simulink library "lib_controls"  (Simulink 7.9)
settings: Solver=ode45  SolverMode=SingleTasking  StartTime=0.0  StopTime=10.0  RelTol=1e-3
undefined symbols (not defined in the file): amb_tmp, cs_charge_deplete_bool, cs_charge_pwr, cs_charge_trq, cs_clt_tmp, cs_decel_fc_off, cs_decel_regen_threshold, cs_dl_assist_trq_threshold, cs_dl_regen_trq_threshold, cs_electric_decel_spd, cs_electric_launch_spd, cs_electric_launch_spd_hi, cs_electric_launch_spd_lo, cs_eng_min_spd, cs_eng_on_soc, cs_fc_init_state, cs_fc_max_pwr_frac, cs_fc_min_pwr_frac, cs_fc_on, cs_fc_pwr_opt, cs_fc_spd_opt, cs_fuzzy_fuel_mode, cs_hi_soc, cs_hi_trq_frac, cs_lo_soc, cs_lo_trq_frac, cs_max_gc_spd, cs_max_pwr, cs_max_pwr_fall_rate, cs_max_pwr_rise_rate, cs_mc_assist_max_frac, cs_mc_assist_min_frac, cs_mc_assist_slope, cs_mc_regen_max_frac, cs_mc_regen_min_frac, cs_mc_regen_slope, cs_mean_eff, cs_mean_eff_bool, cs_min_gc_spd, cs_min_off_time, cs_min_pwr, cs_min_trq_frac, cs_mph_avg_time, cs_off_trq_frac, cs_plot_output, cs_pwr, cs_regen_avg_time, cs_scale_factor, cs_shutoff, cs_soc_range, cs_spd, cs_target_soc, cs_trq_to_soc_factor, cvt_locus_pwr, cvt_locus_spd, cyc_mph, enable_sim_stop_distance, enable_sim_stop_max_spd, enable_sim_stop_speed, enable_sim_stop_time ... (+110)
libraries: lib_controls x124, simulink3 x18, lib_etc x1
(part 4 of 17)

== system lib_controls/<vc> conv auto Saber custom/engine control ==
  shifting : Inport
  clutch state : Inport  Port=2
  fc_spd_out_r : Inport  Port=3
  v_ave_req : Inport  Port=4
  Block NOTES : Subsystem
      mask Display: disp('Block\nNOTES')
  Constant : Constant  Value=1.1
  Constant1 : Constant  Value=vc_idle_bool
  Constant2 : Constant  Value=vc_launch_spd
  Constant3 : Constant
  Constant4 : Constant  Value=0
  Constant5 : Constant  Value=0
  Constant6 : Constant  Value=0
  Logical Operator1 : Logic
  Logical Operator2 : Logic  Operator=OR
  Logical Operator3 : Logic  Operator=OR
  Logical Operator7 : Logic
  Logical Operator8 : Logic  Inputs=3
  Memory : Memory
  Saturation : Saturate  UpperLimit=max(fc_map_spd)*fc_spd_scale  LowerLimit=vc_idle_spd*vc_idle_bool
  Switch : Switch  Threshold=eps  SaturateOnIntegerOverflow=on  InputSameDT=on
  Switch1 : Switch  Threshold=eps  SaturateOnIntegerOverflow=on  InputSameDT=on
  clutch disengaged : RelationalOperator  Operator===  InputSameDT=on
  clutch slipping or engaged : RelationalOperator  Operator=>  InputSameDT=on
  key_on : Subsystem  mask(Repeating table){@1=vc_key_on(:,1), @2=vc_key_on(:,2)}
      mask prompts: @1 "Time values:"; @2 "Output values:"
      mask help:
      | Repeating table.
      | Enter values of time and output for first cycle.
      mask init:
      | period = max(@1); t = @1; y = @2;
      mask Help: Repeats cycle given in table. Time values should be monotonically increasing.
  moving next time : RelationalOperator  Operator=>  InputSameDT=on
  not moving : RelationalOperator  Operator===  InputSameDT=on
  repeated cycle:  speed required at end of NEXT step : Subsystem  mask(Forward looking repeating table){t=cyc_mph(:,1), y=cyc_mph(:,2)}
      mask prompts: t "Time values:"; y "Output values:"
      mask help:
      | Forward looking repeating table.
      | Enter values of time and output for first cycle.
      mask init:
      | period = max(t);
      mask Help: Repeats cycle given in table with a one time step forward offset. Time values should be monotonically increasing.
  engine on : Outport
  spd command  (rad/s) : Outport  Port=2
  key on : Outport  Port=3
  wires:
  clutch state/1 -> clutch slipping or engaged/1, clutch disengaged/1
  Constant/1 -> clutch slipping or engaged/2
  Constant1/1 -> Logical Operator2/2
  clutch slipping or engaged/1 -> Logical Operator2/1
  Logical Operator1/1 -> Logical Operator3/1
  Logical Operator3/1 -> Switch1/2, Memory/1, engine on/1
  Logical Operator2/1 -> Logical Operator1/2
  Constant3/1 -> clutch disengaged/2
  v_ave_req/1 -> not moving/1
  Constant4/1 -> not moving/2
  clutch disengaged/1 -> Logical Operator8/1
  not moving/1 -> Logical Operator8/2
  moving next time/1 -> Logical Operator8/3
  shifting/1 -> Logical Operator7/1
  Logical Operator7/1 -> Logical Operator3/2
  Memory/1 -> Logical Operator7/2
  repeated cycle:  speed required at end of NEXT step/1(out_1) -> moving next time/1
  Constant5/1 -> moving next time/2
  Switch/1 -> Saturation/1
  Constant2/1 -> Switch/1
  fc_spd_out_r/1 -> Switch/3
  Logical Operator8/1 -> Switch/2
  Constant6/1 -> Switch1/3
  Switch1/1 -> spd command  (rad/s)/1
  Saturation/1 -> Switch1/1
  key_on/1(out_1) -> Logical Operator1/1, key on/1

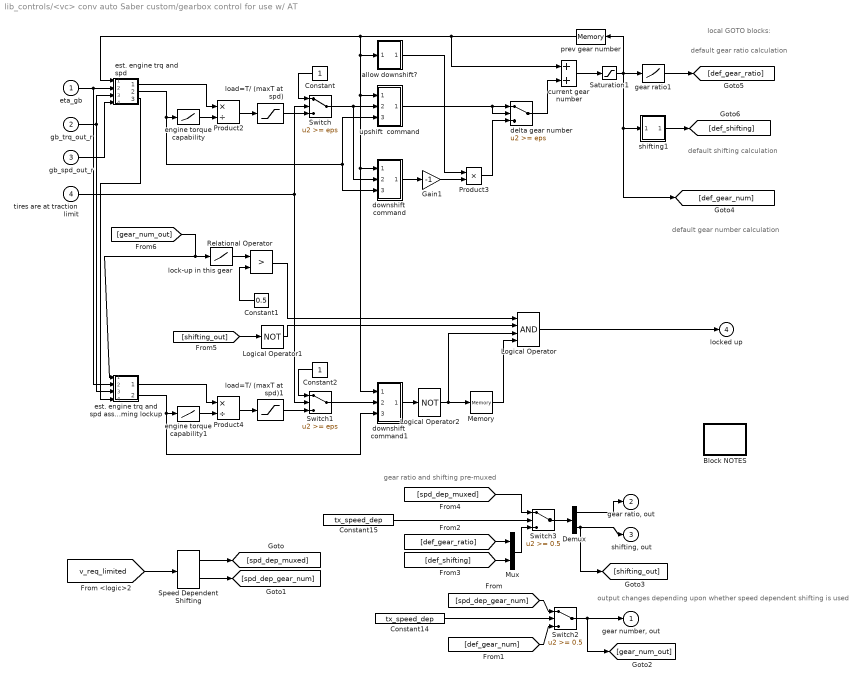
== system lib_controls/<vc> conv auto Saber custom/gearbox control for use w/ AT ==
  note: gear ratio and shifting pre-muxed
  note: output changes depending
      | upon whether speed
      | dependent shifting is used
  note: default gear number
      | calculation
  note: default shifting
      | calculation
  note: default gear ratio
      | calculation
  note: local GOTO blocks:
  eta_gb : Inport
  gb_trq_out_r : Inport  Port=2
  gb_spd_out_r : Inport  Port=3
  tires are at traction limit : Inport  Port=4
  Block NOTES : Subsystem
      mask Display: disp('Block\nNOTES')
  Constant : Constant
  Constant1 : Constant  Value=0.5
  Constant14 : Constant  Value=tx_speed_dep
  Constant15 : Constant  Value=tx_speed_dep
  Constant2 : Constant
  Demux : Demux  Outputs=2
  Gain1 : Gain  Gain=-1  SaturateOnIntegerOverflow=on  OutDataTypeStr=Inherit: Same as input  ParamDataTypeStr=Inherit: Same as input
  Logical Operator : Logic  Inputs=4
  Logical Operator1 : Logic  Operator=NOT  Inputs=1
  Logical Operator2 : Logic  Operator=NOT  Inputs=1
  Memory : Memory
  Mux : Mux  Inputs=2
  Product2 : Product  Inputs=*/  SaturateOnIntegerOverflow=on  RndMeth=Zero  InputSameDT=on  OutDataTypeStr=Inherit: Same as first input
  Product3 : Product  SaturateOnIntegerOverflow=on  RndMeth=Zero  InputSameDT=on  OutDataTypeStr=Inherit: Same as first input
  Product4 : Product  Inputs=*/  SaturateOnIntegerOverflow=on  RndMeth=Zero  InputSameDT=on  OutDataTypeStr=Inherit: Same as first input
  Relational Operator : RelationalOperator  Operator=>  InputSameDT=on
  Saturation1 : Saturate  UpperLimit=gb_gears_num  LowerLimit=1
  Speed Dependent Shifting : lib_controls/SubSystem/Speed Dependent Shifting
      settings: RTWFcnNameOpts=Auto  RTWFileNameOpts=Auto
  Switch : Switch  Threshold=eps  SaturateOnIntegerOverflow=on  InputSameDT=on
  Switch1 : Switch  Threshold=eps  SaturateOnIntegerOverflow=on  InputSameDT=on
  Switch2 : Switch  Threshold=0.5  SaturateOnIntegerOverflow=on  InputSameDT=on
  Switch3 : Switch  Threshold=0.5  SaturateOnIntegerOverflow=on  InputSameDT=on
  allow downshift? : Subsystem
  current gear number : Sum  SaturateOnIntegerOverflow=on  InputSameDT=on  OutDataTypeStr=Inherit: Same as first input
  delta gear number : Switch  Threshold=eps  SaturateOnIntegerOverflow=on  InputSameDT=on
  downshift  command : Subsystem
  downshift  command1 : Subsystem
  engine torque capability : Lookup  InputValues=fc_map_spd*fc_spd_scale  Table=fc_max_trq*fc_trq_scale+eps  SaturateOnIntegerOverflow=on
  engine torque capability1 : Lookup  InputValues=fc_map_spd*fc_spd_scale  Table=fc_max_trq*fc_trq_scale+eps  SaturateOnIntegerOverflow=on
  est. engine trq and spd : Subsystem
  est. engine trq and spd assuming lockup : Subsystem
  gear ratio1 : Lookup  InputValues=[1:length(gb_ratio)]  Table=gb_ratio  SaturateOnIntegerOverflow=on
  load=T/ (maxT at spd) : Saturate  UpperLimit=1  LowerLimit=-1
  load=T/ (maxT at spd)1 : Saturate  UpperLimit=1  LowerLimit=-1
  lock-up in this gear : Lookup  InputValues=[1:length(htc_lockup)]  Table=htc_lockup  SaturateOnIntegerOverflow=on
  prev gear number : Memory  X0=gb_num_init
  shifting1 : Subsystem
  upshift  command : Subsystem
  "gear number, out" : Outport  InitialOutput=0
  "gear ratio, out" : Outport  Port=2  InitialOutput=0
  "shifting, out" : Outport  Port=3  InitialOutput=0
  locked up : Outport  Port=4  InitialOutput=0
  wires:
  downshift  command1/1(command) -> Logical Operator2/1
  load=T/ (maxT at spd)1/1 -> Switch1/3
  Memory/1 -> Logical Operator/4
  Switch1/1 -> downshift  command1/2(engine load)
  Logical Operator/1 -> locked up/1
  Gain1/1 -> Product3/2
  upshift  command/1(command) -> delta gear number/1, delta gear number/2
  Switch/1 -> upshift  command/2(engine load), downshift  command/2(engine load)
  Logical Operator2/1 -> Memory/1, Logical Operator/3
  est. engine trq and spd assuming lockup/2(est eng spd (rad/s)) -> downshift  command1/3(engine speed), engine torque capability1/1
  est. engine trq and spd/3(gb_spd_in_est (rad/s)1) -> est. engine trq and spd assuming lockup/4(gb_spd_in_est)
  tires are at traction limit/1 -> Switch/2, Switch1/2
  gb_trq_out_r/1 -> est. engine trq and spd assuming lockup/3(gb_trq_out_r), est. engine trq and spd/3(gb_trq_out_r)
  eta_gb/1 -> est. engine trq and spd assuming lockup/2(" prev eta_gb"), est. engine trq and spd/2(" prev eta_gb")
  est. engine trq and spd assuming lockup/1(est eng trq (Nm)) -> Product4/1
  engine torque capability1/1 -> Product4/2
  Product4/1 -> load=T/ (maxT at spd)1/1
  Constant2/1 -> Switch1/1
  Logical Operator1/1 -> Logical Operator/2
  downshift  command/1(command) -> Gain1/1
  load=T/ (maxT at spd)/1 -> Switch/3
  est. engine trq and spd/1(est eng trq (Nm)) -> Product2/1
  engine torque capability/1 -> Product2/2
  current gear number/1 -> Saturation1/1
  Product3/1 -> delta gear number/3
  allow downshift?/1(allow shift) -> Product3/1
  delta gear number/1 -> current gear number/2
  Product2/1 -> load=T/ (maxT at spd)/1
  Constant/1 -> Switch/1
  Saturation1/1 -> gear ratio1/1, prev gear number/1, shifting1/1(gear number), [def_gear_num]
  prev gear number/1 -> est. engine trq and spd/1(prev gear number), allow downshift?/1(prev gearnum), downshift  command1/1(prev gear number), downshift  command/1(prev gear number), upshift  command/1(prev gear number), current gear number/1
  gb_spd_out_r/1 -> est. engine trq and spd/4(gb_spd_out_r)
  est. engine trq and spd/2(est eng spd (rad/s)) -> engine torque capability/1, upshift  command/3(engine speed), downshift  command/3(engine speed)
  Constant15/1 -> Switch3/2
  [spd_dep_muxed] -> Switch3/1
  Mux/1 -> Switch3/3
  [def_gear_ratio] -> Mux/1
  [def_shifting] -> Mux/2
  Switch3/1 -> Demux/1
  Demux/1 -> "gear ratio, out"/1
  Constant14/1 -> Switch2/2
  [spd_dep_gear_num] -> Switch2/1
  [def_gear_num] -> Switch2/3
  [v_req_limited] -> Speed Dependent Shifting/1
  Speed Dependent Shifting/1 -> [spd_dep_muxed]
  Speed Dependent Shifting/2 -> [spd_dep_gear_num]
  Switch2/1 -> "gear number, out"/1, [gear_num_out]
  Demux/2 -> "shifting, out"/1, [shifting_out]
  [shifting_out] -> Logical Operator1/1
  [gear_num_out] -> lock-up in this gear/1, est. engine trq and spd assuming lockup/1(new gear number)
  Relational Operator/1 -> Logical Operator/1
  lock-up in this gear/1 -> Relational Operator/1
  Constant1/1 -> Relational Operator/2
  gear ratio1/1 -> [def_gear_ratio]
  shifting1/1(out_1) -> [def_shifting]

== system lib_controls/<vc> conv cvt/clutch control ==
  shifting : Inport
  gb_trq_in_r : Inport  Port=2
  gb_spd_in_r : Inport  Port=3
  Block NOTES : Subsystem
      mask Display: disp('Block\nNOTES')
  Constant : Constant  Value=1e-3
  Constant1 : Constant  Value=vc_clutch_bool
  Constant2 : Constant  Value=vc_idle_spd
  Constant3 : Constant  Value=1e-3
  Constant4 : Constant  Value=vc_launch_spd
  Constant5 : Constant  Value=2.5
  Fcn: 1 if clutch disengaged 2 if clutch slipping 3 if clutch engaged : Fcn  Expr=u[1]+2*u[2]*(1-u[1])*(1-u[3])+3*u[3]*(1-u[1])
  Logical Operator : Logic
  Logical Operator1 : Logic  Operator=OR
  Memory : Memory  X0=1+(2*(cyc_mph(1,2)>0))
  Mux : Mux  Inputs=3
  Relational Operator : RelationalOperator  Operator=<=  InputSameDT=on
  Relational Operator1 : RelationalOperator  Operator=<  InputSameDT=on
  Relational Operator2 : RelationalOperator  Operator=>  InputSameDT=on
  Relational Operator3 : RelationalOperator  Operator=<  InputSameDT=on
  clutch disengaged : Logic  Operator=OR
  clutch engaged : Logic  Operator=NOR
  clutch slipping : Logic  Inputs=3
  clutch was NOT fully engaged during last time step : RelationalOperator  Operator=<  InputSameDT=on
  clutch state : Outport
  wires:
  Relational Operator1/1 -> Logical Operator1/2
  Constant2/1 -> Relational Operator1/2
  gb_spd_in_r/1 -> Relational Operator1/1, Relational Operator3/1
  Mux/1 -> Fcn: 1 if clutch disengaged 2 if clutch slipping 3 if clutch engaged/1
  clutch engaged/1 -> Mux/3
  clutch disengaged/1 -> clutch engaged/1, Mux/1
  Fcn: 1 if clutch disengaged 2 if clutch slipping 3 if clutch engaged/1 -> clutch state/1, Memory/1
  Constant3/1 -> Relational Operator2/2
  Relational Operator2/1 -> clutch slipping/1
  clutch slipping/1 -> clutch engaged/2, Mux/2
  Constant4/1 -> Relational Operator3/2
  Relational Operator3/1 -> clutch slipping/2
  Memory/1 -> clutch was NOT fully engaged during last time step/1
  Constant5/1 -> clutch was NOT fully engaged during last time step/2
  clutch was NOT fully engaged during last time step/1 -> clutch slipping/3
  Constant1/1 -> Logical Operator1/1
  Constant/1 -> Relational Operator/2
  Relational Operator/1 -> Logical Operator/1
  Logical Operator1/1 -> Logical Operator/2
  gb_trq_in_r/1 -> Relational Operator/1, Relational Operator2/1
  Logical Operator/1 -> clutch disengaged/2
  shifting/1 -> clutch disengaged/1

== system lib_controls/<vc> conv cvt/config traction control ==
  time-average vehicle speed  req'd (m/s) : Inport
  vehicle speed at beginning of time  step (m/s) : Inport  Port=2
  total tractive force req'd (N) : Inport  Port=3
  traction control 2 axle : lib_controls/SubSystem/traction control 2 axle
  req'd force (N) : Outport
  req'd speed (m/s) : Outport  Port=2
  weight on front axle (N) : Outport  Port=3
  weight on rear axle (N) : Outport  Port=4
  front/total  traction ratio : Outport  Port=5
  wires:
  time-average vehicle speed  req'd (m/s)/1 -> traction control 2 axle/1
  vehicle speed at beginning of time  step (m/s)/1 -> traction control 2 axle/2
  total tractive force req'd (N)/1 -> traction control 2 axle/3
  traction control 2 axle/1 -> req'd force (N)/1
  traction control 2 axle/2 -> req'd speed (m/s)/1
  traction control 2 axle/3 -> weight on front axle (N)/1
  traction control 2 axle/4 -> weight on rear axle (N)/1
  traction control 2 axle/5 -> front/total  traction ratio/1

== system lib_controls/<vc> conv cvt/cvt control ==
  cvt_trq_out_r : Inport
  cvt_spd_out_r : Inport  Port=2
  prev. Pout/Pin : Inport  Port=3
  tires are at traction limit : Inport  Port=4
  Block NOTES : Subsystem
      mask Display: disp('Block\nNOTES')
  Constant1 : Constant  Value=eps
  Constant2 : Constant  Value=eps
  Product : Product  Inputs=**/  SaturateOnIntegerOverflow=on  RndMeth=Zero  InputSameDT=on  OutDataTypeStr=Inherit: Same as first input
  Product1 : Product  Inputs=*/  SaturateOnIntegerOverflow=on  RndMeth=Zero  InputSameDT=on  OutDataTypeStr=Inherit: Same as first input
  Saturation1 : Saturate  UpperLimit=max(gb_ratio)  LowerLimit=min(gb_ratio)
  Saturation2 : Saturate  UpperLimit=max(cvt_locus_pwr)*fc_trq_scale*fc_spd_scale  LowerLimit=min(cvt_locus_pwr)*fc_trq_scale*fc_spd_scale
  Sum : Sum  SaturateOnIntegerOverflow=on  InputSameDT=on  OutDataTypeStr=Inherit: Same as first input
  Terminator : Terminator
  desired engine speed : Lookup  InputValues=cvt_locus_pwr*fc_trq_scale*fc_spd_scale  Table=cvt_locus_spd*fc_spd_scale+eps  SaturateOnIntegerOverflow=on
  est. engine power : Sum  SaturateOnIntegerOverflow=on  InputSameDT=on  OutDataTypeStr=Inherit: Same as first input
  output speed : Sum  SaturateOnIntegerOverflow=on  InputSameDT=on  OutDataTypeStr=Inherit: Same as first input
  "pulley ratio " : Outport  InitialOutput=0
  wires:
  output speed/1 -> Product1/2
  Constant1/1 -> output speed/2
  Product/1 -> est. engine power/2
  desired engine speed/1 -> Product1/1
  est. engine power/1 -> Saturation2/1
  Product1/1 -> Saturation1/1
  Saturation2/1 -> desired engine speed/1
  [acc_mech_pwr_est] -> est. engine power/1
  cvt_spd_out_r/1 -> output speed/1, Product/2
  cvt_trq_out_r/1 -> Product/1
  prev. Pout/Pin/1 -> Sum/1
  Sum/1 -> Product/3
  Constant2/1 -> Sum/2
  tires are at traction limit/1 -> Terminator/1
  Saturation1/1 -> "pulley ratio "/1

== system lib_controls/<vc> conv cvt/engine control ==
  clutch state : Inport
  shifting : Inport  Port=2
  fc_spd_out_r : Inport  Port=3
  v_ave_req : Inport  Port=4
  Block NOTES : Subsystem
      mask Display: disp('Block\nNOTES')
  Constant : Constant  Value=1.1
  Constant1 : Constant  Value=vc_idle_bool
  Constant2 : Constant  Value=vc_launch_spd
  Constant3 : Constant
  Constant4 : Constant  Value=0
  Constant5 : Constant  Value=0
  Constant6 : Constant  Value=0
  Logical Operator1 : Logic
  Logical Operator2 : Logic  Operator=OR
  Logical Operator3 : Logic  Operator=OR
  Logical Operator7 : Logic
  Logical Operator8 : Logic  Inputs=3
  Memory : Memory
  Saturation : Saturate  UpperLimit=max(fc_map_spd)*fc_spd_scale  LowerLimit=vc_idle_spd*vc_idle_bool
  Switch : Switch  Threshold=eps  SaturateOnIntegerOverflow=on  InputSameDT=on
  Switch1 : Switch  Threshold=eps  SaturateOnIntegerOverflow=on  InputSameDT=on
  clutch disengaged : RelationalOperator  Operator===  InputSameDT=on
  clutch slipping or engaged : RelationalOperator  Operator=>  InputSameDT=on
  key_on : Subsystem  mask(Repeating table){t=vc_key_on(:,1), y=vc_key_on(:,2)}
      mask prompts: t "Time values:"; y "Output values:"
      mask help:
      | Repeating table.
      | Enter values of time and output for first cycle.
      mask init:
      | period = max(t);
      mask Help: Repeats cycle given in table. Time values should be monotonically increasing.
  moving next time : RelationalOperator  Operator=>  InputSameDT=on
  not moving : RelationalOperator  Operator===  InputSameDT=on
  repeated cycle:  speed required at end of NEXT step : Subsystem  mask(Forward looking repeating table){t=cyc_mph(:,1), y=cyc_mph(:,2)}
      mask prompts: t "Time values:"; y "Output values:"
      mask help:
      | Forward looking repeating table.
      | Enter values of time and output for first cycle.
      mask init:
      | period = max(t);
      mask Help: Repeats cycle given in table with a one time step forward offset. Time values should be monotonically increasing.
  engine on : Outport
  spd command  (rad/s) : Outport  Port=2
  key on : Outport  Port=3
  wires:
  clutch slipping or engaged/1 -> Logical Operator2/1
  Constant/1 -> clutch slipping or engaged/2
  Constant1/1 -> Logical Operator2/2
  clutch state/1 -> clutch slipping or engaged/1, clutch disengaged/1
  Logical Operator1/1 -> Logical Operator3/1
  Logical Operator3/1 -> Switch1/2, Memory/1, engine on/1
  Logical Operator2/1 -> Logical Operator1/2
  key_on/1(out_1) -> Logical Operator1/1, key on/1
  Memory/1 -> Logical Operator7/2
  shifting/1 -> Logical Operator7/1
  Logical Operator7/1 -> Logical Operator3/2
  Constant6/1 -> Switch1/3
  Switch1/1 -> spd command  (rad/s)/1
  Saturation/1 -> Switch1/1
  Constant3/1 -> clutch disengaged/2
  v_ave_req/1 -> not moving/1
  Switch/1 -> Saturation/1
  Constant4/1 -> not moving/2
  repeated cycle:  speed required at end of NEXT step/1(out_1) -> moving next time/1
  Constant5/1 -> moving next time/2
  clutch disengaged/1 -> Logical Operator8/1
  not moving/1 -> Logical Operator8/2
  moving next time/1 -> Logical Operator8/3
  Constant2/1 -> Switch/1
  fc_spd_out_r/1 -> Switch/3
  Logical Operator8/1 -> Switch/2

== system lib_controls/<vc> conv cvt Saber custom/clutch control ==
  shifting : Inport
  gb_trq_in_r : Inport  Port=2
  gb_spd_in_r : Inport  Port=3
  Block NOTES : Subsystem
      mask Display: disp('Block\nNOTES')
  Constant : Constant  Value=1e-3
  Constant1 : Constant  Value=vc_clutch_bool
  Constant2 : Constant  Value=vc_idle_spd
  Constant3 : Constant  Value=1e-3
  Constant4 : Constant  Value=vc_launch_spd
  Constant5 : Constant  Value=2.5
  Fcn: 1 if clutch disengaged 2 if clutch slipping 3 if clutch engaged : Fcn  Expr=u[1]+2*u[2]*(1-u[1])*(1-u[3])+3*u[3]*(1-u[1])
  Logical Operator : Logic
  Logical Operator1 : Logic  Operator=OR
  Memory : Memory  X0=1+(2*(cyc_mph(1,2)>0))
  Mux : Mux  Inputs=3
  Relational Operator : RelationalOperator  Operator=<=  InputSameDT=on
  Relational Operator1 : RelationalOperator  Operator=<  InputSameDT=on
  Relational Operator2 : RelationalOperator  Operator=>  InputSameDT=on
  Relational Operator3 : RelationalOperator  Operator=<  InputSameDT=on
  clutch disengaged : Logic  Operator=OR
  clutch engaged : Logic  Operator=NOR
  clutch slipping : Logic  Inputs=3
  clutch was NOT fully engaged during last time step : RelationalOperator  Operator=<  InputSameDT=on
  clutch state : Outport
  wires:
  shifting/1 -> clutch disengaged/1
  Logical Operator/1 -> clutch disengaged/2
  gb_trq_in_r/1 -> Relational Operator2/1, Relational Operator/1
  Logical Operator1/1 -> Logical Operator/2
  Relational Operator/1 -> Logical Operator/1
  Constant/1 -> Relational Operator/2
  Constant1/1 -> Logical Operator1/1
  clutch was NOT fully engaged during last time step/1 -> clutch slipping/3
  Constant5/1 -> clutch was NOT fully engaged during last time step/2
  Memory/1 -> clutch was NOT fully engaged during last time step/1
  Relational Operator3/1 -> clutch slipping/2
  Constant4/1 -> Relational Operator3/2
  clutch slipping/1 -> Mux/2, clutch engaged/2
  Relational Operator2/1 -> clutch slipping/1
  Constant3/1 -> Relational Operator2/2
  Fcn: 1 if clutch disengaged 2 if clutch slipping 3 if clutch engaged/1 -> Memory/1, clutch state/1
  clutch disengaged/1 -> Mux/1, clutch engaged/1
  clutch engaged/1 -> Mux/3
  Mux/1 -> Fcn: 1 if clutch disengaged 2 if clutch slipping 3 if clutch engaged/1
  gb_spd_in_r/1 -> Relational Operator3/1, Relational Operator1/1
  Constant2/1 -> Relational Operator1/2
  Relational Operator1/1 -> Logical Operator1/2

== system lib_controls/<vc> conv cvt Saber custom/config traction control ==
  time-average vehicle speed  req'd (m/s) : Inport
  vehicle speed at beginning of time  step (m/s) : Inport  Port=2
  total tractive force req'd (N) : Inport  Port=3
  traction control 2 axle : lib_controls/SubSystem/traction control 2 axle
      settings: RTWFcnNameOpts=Auto  RTWFileNameOpts=Auto
  req'd force (N) : Outport
  req'd speed (m/s) : Outport  Port=2
  weight on front axle (N) : Outport  Port=3
  weight on rear axle (N) : Outport  Port=4
  front/total  traction ratio : Outport  Port=5
  wires:
  time-average vehicle speed  req'd (m/s)/1 -> traction control 2 axle/1
  vehicle speed at beginning of time  step (m/s)/1 -> traction control 2 axle/2
  total tractive force req'd (N)/1 -> traction control 2 axle/3
  traction control 2 axle/1 -> req'd force (N)/1
  traction control 2 axle/2 -> req'd speed (m/s)/1
  traction control 2 axle/3 -> weight on front axle (N)/1
  traction control 2 axle/4 -> weight on rear axle (N)/1
  traction control 2 axle/5 -> front/total  traction ratio/1

== system lib_controls/<vc> conv cvt Saber custom/cvt control ==
  cvt_trq_out_r : Inport
  cvt_spd_out_r : Inport  Port=2
  prev. Pout/Pin : Inport  Port=3
  tires are at traction limit : Inport  Port=4
  Block NOTES : Subsystem
      mask Display: disp('Block\nNOTES')
  Constant1 : Constant  Value=eps
  Constant2 : Constant  Value=eps
  Product : Product  Inputs=**/  SaturateOnIntegerOverflow=on  RndMeth=Zero  InputSameDT=on  OutDataTypeStr=Inherit: Same as first input
  Product1 : Product  Inputs=*/  SaturateOnIntegerOverflow=on  RndMeth=Zero  InputSameDT=on  OutDataTypeStr=Inherit: Same as first input
  Saturation1 : Saturate  UpperLimit=max(gb_ratio)  LowerLimit=min(gb_ratio)
  Saturation2 : Saturate  UpperLimit=max(cvt_locus_pwr)*fc_trq_scale*fc_spd_scale  LowerLimit=min(cvt_locus_pwr)*fc_trq_scale*fc_spd_scale
  Sum : Sum  SaturateOnIntegerOverflow=on  InputSameDT=on  OutDataTypeStr=Inherit: Same as first input
  Terminator : Terminator
  accessories (Nm) : lib_controls/<vc> conv Saber custom/gearbox  control/accessories (Nm)
      settings: RTWFcnNameOpts=Auto  RTWFileNameOpts=Auto
  desired engine speed : Lookup  InputValues=cvt_locus_pwr*fc_trq_scale*fc_spd_scale  Table=cvt_locus_spd*fc_spd_scale+eps  SaturateOnIntegerOverflow=on
  est. engine power : Sum  SaturateOnIntegerOverflow=on  InputSameDT=on  OutDataTypeStr=Inherit: Same as first input
  output speed : Sum  SaturateOnIntegerOverflow=on  InputSameDT=on  OutDataTypeStr=Inherit: Same as first input
  "pulley ratio " : Outport  InitialOutput=0
  wires:
  Saturation1/1 -> "pulley ratio "/1
  tires are at traction limit/1 -> Terminator/1
  Constant2/1 -> Sum/2
  Sum/1 -> Product/3
  prev. Pout/Pin/1 -> Sum/1
  cvt_trq_out_r/1 -> Product/1
  cvt_spd_out_r/1 -> output speed/1, Product/2
  accessories (Nm)/1 -> est. engine power/1
  Saturation2/1 -> desired engine speed/1
  Product1/1 -> Saturation1/1
  est. engine power/1 -> Saturation2/1
  desired engine speed/1 -> Product1/1
  Product/1 -> est. engine power/2
  Constant1/1 -> output speed/2
  output speed/1 -> Product1/2

== system lib_controls/<vc> conv cvt Saber custom/engine control ==
  clutch state : Inport
  shifting : Inport  Port=2
  fc_spd_out_r : Inport  Port=3
  v_ave_req : Inport  Port=4
  Block NOTES : Subsystem
      mask Display: disp('Block\nNOTES')
  Constant : Constant  Value=1.1
  Constant1 : Constant  Value=vc_idle_bool
  Constant2 : Constant  Value=vc_launch_spd
  Constant3 : Constant
  Constant4 : Constant  Value=0
  Constant5 : Constant  Value=0
  Constant6 : Constant  Value=0
  Logical Operator1 : Logic
  Logical Operator2 : Logic  Operator=OR
  Logical Operator3 : Logic  Operator=OR
  Logical Operator7 : Logic
  Logical Operator8 : Logic  Inputs=3
  Memory : Memory
  Saturation : Saturate  UpperLimit=max(fc_map_spd)*fc_spd_scale  LowerLimit=vc_idle_spd*vc_idle_bool
  Switch : Switch  Threshold=eps  SaturateOnIntegerOverflow=on  InputSameDT=on
  Switch1 : Switch  Threshold=eps  SaturateOnIntegerOverflow=on  InputSameDT=on
  clutch disengaged : RelationalOperator  Operator===  InputSameDT=on
  clutch slipping or engaged : RelationalOperator  Operator=>  InputSameDT=on
  key_on : Subsystem  mask(Repeating table){@1=vc_key_on(:,1), @2=vc_key_on(:,2)}
      mask prompts: @1 "Time values:"; @2 "Output values:"
      mask help:
      | Repeating table.
      | Enter values of time and output for first cycle.
      mask init:
      | period = max(@1); t = @1; y = @2;
      mask Help: Repeats cycle given in table. Time values should be monotonically increasing.
  moving next time : RelationalOperator  Operator=>  InputSameDT=on
  not moving : RelationalOperator  Operator===  InputSameDT=on
  repeated cycle:  speed required at end of NEXT step : Subsystem  mask(Forward looking repeating table){t=cyc_mph(:,1), y=cyc_mph(:,2)}
      mask prompts: t "Time values:"; y "Output values:"
      mask help:
      | Forward looking repeating table.
      | Enter values of time and output for first cycle.
      mask init:
      | period = max(t);
      mask Help: Repeats cycle given in table with a one time step forward offset. Time values should be monotonically increasing.
  engine on : Outport
  spd command  (rad/s) : Outport  Port=2
  key on : Outport  Port=3
  wires:
  Logical Operator8/1 -> Switch/2
  fc_spd_out_r/1 -> Switch/3
  Constant2/1 -> Switch/1
  moving next time/1 -> Logical Operator8/3
  not moving/1 -> Logical Operator8/2
  clutch disengaged/1 -> Logical Operator8/1
  Constant5/1 -> moving next time/2
  repeated cycle:  speed required at end of NEXT step/1(out_1) -> moving next time/1
  Constant4/1 -> not moving/2
  Switch/1 -> Saturation/1
  v_ave_req/1 -> not moving/1
  Constant3/1 -> clutch disengaged/2
  Saturation/1 -> Switch1/1
  Switch1/1 -> spd command  (rad/s)/1
  Constant6/1 -> Switch1/3
  Logical Operator7/1 -> Logical Operator3/2
  shifting/1 -> Logical Operator7/1
  Memory/1 -> Logical Operator7/2
  key_on/1(out_1) -> key on/1, Logical Operator1/1
  Logical Operator2/1 -> Logical Operator1/2
  Logical Operator3/1 -> engine on/1, Memory/1, Switch1/2
  Logical Operator1/1 -> Logical Operator3/1
  clutch state/1 -> clutch disengaged/1, clutch slipping or engaged/1
  Constant1/1 -> Logical Operator2/2
  Constant/1 -> clutch slipping or engaged/2
  clutch slipping or engaged/1 -> Logical Operator2/1

== system lib_controls/<vc> ev/config traction control ==
  time-average vehicle speed  req'd (m/s) : Inport
  vehicle speed at beginning of time  step (m/s) : Inport  Port=2
  total tractive force req'd (N) : Inport  Port=3
  traction control 2 axle : lib_controls/SubSystem/traction control 2 axle
      settings: RTWFcnNameOpts=Auto  RTWFileNameOpts=Auto
  req'd force (N) : Outport
  req'd speed (m/s) : Outport  Port=2
  weight on front axle (N) : Outport  Port=3
  weight on rear axle (N) : Outport  Port=4
  front/total  traction ratio : Outport  Port=5
  wires:
  time-average vehicle speed  req'd (m/s)/1 -> traction control 2 axle/1
  vehicle speed at beginning of time  step (m/s)/1 -> traction control 2 axle/2
  total tractive force req'd (N)/1 -> traction control 2 axle/3
  traction control 2 axle/1 -> req'd force (N)/1
  traction control 2 axle/2 -> req'd speed (m/s)/1
  traction control 2 axle/3 -> weight on front axle (N)/1
  traction control 2 axle/4 -> weight on rear axle (N)/1
  traction control 2 axle/5 -> front/total  traction ratio/1

== system lib_controls/<vc> ev/gearbox control for series  HV and EV ==
  note: default gear number
      | calculation
  note: default shifting
      | calculation
  note: default gear ratio
      | calculation
  note: local GOTO blocks:
  gb_trq_out_r : Inport
  gb_spd_out_r : Inport  Port=2
  prev. Pout/Pin : Inport  Port=3
  tires are at traction limit : Inport  Port=4
  Block NOTES : Subsystem
      mask Display: disp('Block\nNOTES')
  Constant : Constant
  Constant14 : Constant  Value=tx_speed_dep
  Constant15 : Constant  Value=tx_speed_dep
  Demux : Demux  Outputs=2
  Fcn : Fcn  Expr=1/u
  Fcn1 : Fcn  Expr=1/u
  Gain1 : Gain  Gain=-1  SaturateOnIntegerOverflow=on  OutDataTypeStr=Inherit: Same as input  ParamDataTypeStr=Inherit: Same as input
  MOTOR torque capability : Lookup  InputValues=mc_map_spd*mc_spd_scale  Table=mc_max_trq*mc_trq_scale+eps  SaturateOnIntegerOverflow=on
  Mux : Mux  Inputs=2
  Product2 : Product  Inputs=*/  SaturateOnIntegerOverflow=on  RndMeth=Zero  InputSameDT=on  OutDataTypeStr=Inherit: Same as first input
  Product3 : Product  SaturateOnIntegerOverflow=on  RndMeth=Zero  InputSameDT=on  OutDataTypeStr=Inherit: Same as first input
  Rate Limiter : RateLimiter  RisingSlewLimit=1/(gb_shift_delay+eps)  FallingSlewLimit=-1/(gb_shift_delay+eps)
  Saturation : Saturate  UpperLimit=1  LowerLimit=0.2
  Saturation1 : Saturate  UpperLimit=gb_gears_num  LowerLimit=1
  Speed Dependent Shifting : lib_controls/SubSystem/Speed Dependent Shifting
      settings: RTWFcnNameOpts=Auto  RTWFileNameOpts=Auto
  Switch : Switch  Threshold=eps  SaturateOnIntegerOverflow=on  InputSameDT=on
  Switch3 : Switch  Threshold=0.5  SaturateOnIntegerOverflow=on  InputSameDT=on
  Switch4 : Switch  Threshold=0.5  SaturateOnIntegerOverflow=on  InputSameDT=on
  allow downshift? : Subsystem
  current gear number : Sum  SaturateOnIntegerOverflow=on  InputSameDT=on  OutDataTypeStr=Inherit: Same as first input
  delta gear number : Switch  Threshold=eps  SaturateOnIntegerOverflow=on  InputSameDT=on
  downshift  command : Subsystem
  gb_spd_in_r : Product  SaturateOnIntegerOverflow=on  RndMeth=Zero  InputSameDT=on  OutDataTypeStr=Inherit: Same as first input
  gear ratio : Lookup  InputValues=[1:length(gb_ratio)]  Table=gb_ratio  SaturateOnIntegerOverflow=on
  gear ratio1 : Lookup  InputValues=[1:length(gb_ratio)]  Table=gb_ratio  SaturateOnIntegerOverflow=on
  gearbox speed estimator : Subsystem
  load=T/ (maxT at spd) : Saturate  UpperLimit=1  LowerLimit=0
  prev gear number : Memory  X0=1
  prev gear ratio : Memory  X0=gb_ratio(1)
  shifting1 : Subsystem
  upshift  command : Subsystem
  ~gb_trq_in_r : Product  Inputs=3  SaturateOnIntegerOverflow=on  RndMeth=Zero  InputSameDT=on  OutDataTypeStr=Inherit: Same as first input
  "gear number, out" : Outport  InitialOutput=0
  "gear ratio, out" : Outport  Port=2  InitialOutput=0
  "shifting, out" : Outport  Port=3  InitialOutput=0
  wires:
  gearbox speed estimator/1(Out1) -> MOTOR torque capability/1, downshift  command/3(engine speed), upshift  command/3(engine speed)
  gb_spd_in_r/1 -> gearbox speed estimator/1(gb_spd_in_r if no gear change)
  current gear number/1 -> Saturation1/1
  Saturation/1 -> Fcn/1
  prev. Pout/Pin/1 -> Saturation/1
  gb_trq_out_r/1 -> ~gb_trq_in_r/1
  upshift  command/1(command) -> delta gear number/1, delta gear number/2
  gear ratio/1 -> prev gear ratio/1
  Rate Limiter/1 -> gear ratio/1
  gb_spd_out_r/1 -> gb_spd_in_r/1
  downshift  command/1(command) -> Gain1/1
  Gain1/1 -> Product3/2
  Product3/1 -> delta gear number/3
  allow downshift?/1(allow shift) -> Product3/1
  prev gear ratio/1 -> Fcn1/1, gb_spd_in_r/2
  delta gear number/1 -> current gear number/2
  Fcn1/1 -> ~gb_trq_in_r/3
  MOTOR torque capability/1 -> Product2/2
  Product2/1 -> load=T/ (maxT at spd)/1
  ~gb_trq_in_r/1 -> Product2/1
  Fcn/1 -> ~gb_trq_in_r/2
  load=T/ (maxT at spd)/1 -> Switch/3
  tires are at traction limit/1 -> Switch/2
  Constant/1 -> Switch/1
  Switch/1 -> upshift  command/2(engine load), downshift  command/2(engine load)
  Saturation1/1 -> prev gear number/1, gear ratio1/1, shifting1/1(gear number), Rate Limiter/1, [def_gear_num]
  prev gear number/1 -> allow downshift?/1(prev gearnum), upshift  command/1(prev gear number), downshift  command/1(prev gear number), current gear number/1
  gear ratio1/1 -> [def_gear_ratio]
  shifting1/1(out_1) -> [def_shifting]
  Constant14/1 -> Switch3/2
  [def_gear_num] -> Switch3/3
  Constant15/1 -> Switch4/2
  [spd_dep_muxed] -> Switch4/1
  Mux/1 -> Switch4/3
  [def_gear_ratio] -> Mux/1
  [def_shifting] -> Mux/2
  Switch4/1 -> Demux/1
  [spd_dep_gear_num] -> Switch3/1
  [v_req_limited] -> Speed Dependent Shifting/1
  Speed Dependent Shifting/1 -> [spd_dep_muxed]
  Speed Dependent Shifting/2 -> [spd_dep_gear_num]
  Demux/1 -> "gear ratio, out"/1
  Demux/2 -> "shifting, out"/1
  Switch3/1 -> "gear number, out"/1

== system lib_controls/<vc> ev/key_on ==
  Clock : Clock
  Fcn1 : Fcn  Expr=rem(u[1],period)
  Look-Up Table : Lookup  InputValues=t  Table=y  SaturateOnIntegerOverflow=on
  out_1 : Outport  InitialOutput=0
  wires:
  Look-Up Table/1 -> out_1/1
  Clock/1 -> Fcn1/1
  Fcn1/1 -> Look-Up Table/1

== system lib_controls/<vc> ev/motor controller logic ==
  shifting : Inport
  bus voltage : Inport  Port=2
  req'd input power (W) : Inport  Port=3
  req'd output spd (rad/s) : Inport  Port=4
  Abs : Abs  SaturateOnIntegerOverflow=on
  Abs1 : Abs  SaturateOnIntegerOverflow=on
  Block NOTES : Subsystem
      mask Display: disp('Block\nNOTES')
  Constant : Constant  Value=mc_max_crrnt
  Constant1 : Constant  Value=0.001
  Constant2 : Constant  Value=0
  Logical Operator1 : Logic  Operator=NOT  Inputs=1
  Memory : Memory  X0=ess_module_num*mean(ess_voc(:,1))
  MinMax : MinMax  Inputs=2  SaturateOnIntegerOverflow=on  InputSameDT=on
  Product1 : Product  SaturateOnIntegerOverflow=on  RndMeth=Zero  InputSameDT=on  OutDataTypeStr=Inherit: Same as first input
  Relational Operator : RelationalOperator  Operator=<=  InputSameDT=on
  Relational Operator2 : RelationalOperator  Operator===  InputSameDT=on
  Sign : Subsystem
      mask Type: Sign
      mask Description: y = sign(x)
      mask Help: Sign Function:\n\t\t\ty = 1 if x > 0\n\t\t\ty = 0 if x = 0\n\t\t\ty = -1 if x < 0
      mask Display: plot(-50,-50,50,50,[-50,50],[0,0],[0,0],[-50,50],[-40,0],[-30,-30],[0,40],[30,30])
  Switch : Switch  Threshold=eps  SaturateOnIntegerOverflow=on  InputSameDT=on
  current-limited power : Product  SaturateOnIntegerOverflow=on  RndMeth=Zero  InputSameDT=on  OutDataTypeStr=Inherit: Same as first input
  true if motor should be shut down : Logic  Operator=OR
  req'd input power (W)1 : Outport  InitialOutput=0
  tag scope: mc_crrnt_limited=global
  wires:
  Relational Operator2/1 -> [mc_crrnt_limited]
  Logical Operator1/1 -> Switch/2
  Constant2/1 -> Switch/3
  Switch/1 -> req'd input power (W)1/1
  current-limited power/1 -> Switch/1
  Sign/1(out_1) -> current-limited power/2
  MinMax/1 -> current-limited power/1, Relational Operator2/2
  req'd input power (W)/1 -> Abs/1, Sign/1(in_1)
  Constant1/1 -> Relational Operator/2
  Abs1/1 -> Relational Operator/1
  shifting/1 -> true if motor should be shut down/2
  Relational Operator/1 -> true if motor should be shut down/1
  req'd output spd (rad/s)/1 -> Abs1/1
  true if motor should be shut down/1 -> Logical Operator1/1
  bus voltage/1 -> Memory/1
  Constant/1 -> Product1/2
  Abs/1 -> MinMax/2
  Product1/1 -> MinMax/1, Relational Operator2/1
  Memory/1 -> Product1/1

== system lib_controls/<vc> fuel cell/config traction control ==
  time-average vehicle speed  req'd (m/s) : Inport
  vehicle speed at beginning of time  step (m/s) : Inport  Port=2
  total tractive force req'd (N) : Inport  Port=3
  traction control 2 axle : lib_controls/SubSystem/traction control 2 axle
      settings: RTWFcnNameOpts=Auto  RTWFileNameOpts=Auto
  req'd force (N) : Outport
  req'd speed (m/s) : Outport  Port=2
  weight on front axle (N) : Outport  Port=3
  weight on rear axle (N) : Outport  Port=4
  front/total  traction ratio : Outport  Port=5
  wires:
  time-average vehicle speed  req'd (m/s)/1 -> traction control 2 axle/1
  vehicle speed at beginning of time  step (m/s)/1 -> traction control 2 axle/2
  total tractive force req'd (N)/1 -> traction control 2 axle/3
  traction control 2 axle/1 -> req'd force (N)/1
  traction control 2 axle/2 -> req'd speed (m/s)/1
  traction control 2 axle/3 -> weight on front axle (N)/1
  traction control 2 axle/4 -> weight on rear axle (N)/1
  traction control 2 axle/5 -> front/total  traction ratio/1

== system lib_controls/<vc> fuel cell/gearbox control for series  HV and EV ==
  note: default gear number
      | calculation
  note: default shifting
      | calculation
  note: default gear ratio
      | calculation
  note: local GOTO blocks:
  gb_trq_out_r : Inport
  gb_spd_out_r : Inport  Port=2
  prev. Pout/Pin : Inport  Port=3
  tires are at traction limit : Inport  Port=4
  Block NOTES : Subsystem
      mask Display: disp('Block\nNOTES')
  Constant : Constant
  Constant14 : Constant  Value=tx_speed_dep
  Constant15 : Constant  Value=tx_speed_dep
  Demux : Demux  Outputs=2
  Fcn : Fcn  Expr=1/u
  Fcn1 : Fcn  Expr=1/u
  Gain1 : Gain  Gain=-1  SaturateOnIntegerOverflow=on  OutDataTypeStr=Inherit: Same as input  ParamDataTypeStr=Inherit: Same as input
  MOTOR torque capability : Lookup  InputValues=mc_map_spd*mc_spd_scale  Table=mc_max_trq*mc_trq_scale+eps  SaturateOnIntegerOverflow=on
  Mux : Mux  Inputs=2
  Product2 : Product  Inputs=*/  SaturateOnIntegerOverflow=on  RndMeth=Zero  InputSameDT=on  OutDataTypeStr=Inherit: Same as first input
  Product3 : Product  SaturateOnIntegerOverflow=on  RndMeth=Zero  InputSameDT=on  OutDataTypeStr=Inherit: Same as first input
  Rate Limiter : RateLimiter  RisingSlewLimit=1/(gb_shift_delay+eps)  FallingSlewLimit=-1/(gb_shift_delay+eps)
  Saturation : Saturate  UpperLimit=1  LowerLimit=0.2
  Saturation1 : Saturate  UpperLimit=gb_gears_num  LowerLimit=1
  Speed Dependent Shifting : lib_controls/SubSystem/Speed Dependent Shifting
      settings: RTWFcnNameOpts=Auto  RTWFileNameOpts=Auto
  Switch : Switch  Threshold=eps  SaturateOnIntegerOverflow=on  InputSameDT=on
  Switch3 : Switch  Threshold=0.5  SaturateOnIntegerOverflow=on  InputSameDT=on
  Switch4 : Switch  Threshold=0.5  SaturateOnIntegerOverflow=on  InputSameDT=on
  allow downshift? : Subsystem
  current gear number : Sum  SaturateOnIntegerOverflow=on  InputSameDT=on  OutDataTypeStr=Inherit: Same as first input
  delta gear number : Switch  Threshold=eps  SaturateOnIntegerOverflow=on  InputSameDT=on
  downshift  command : Subsystem
  gb_spd_in_r : Product  SaturateOnIntegerOverflow=on  RndMeth=Zero  InputSameDT=on  OutDataTypeStr=Inherit: Same as first input
  gear ratio : Lookup  InputValues=[1:length(gb_ratio)]  Table=gb_ratio  SaturateOnIntegerOverflow=on
  gear ratio1 : Lookup  InputValues=[1:length(gb_ratio)]  Table=gb_ratio  SaturateOnIntegerOverflow=on
  gearbox speed estimator : Subsystem
  load=T/ (maxT at spd) : Saturate  UpperLimit=1  LowerLimit=0
  prev gear number : Memory  X0=1
  prev gear ratio : Memory  X0=gb_ratio(1)
  shifting1 : Subsystem
  upshift  command : Subsystem
  ~gb_trq_in_r : Product  Inputs=3  SaturateOnIntegerOverflow=on  RndMeth=Zero  InputSameDT=on  OutDataTypeStr=Inherit: Same as first input
  "gear number, out" : Outport  InitialOutput=0
  "gear ratio, out" : Outport  Port=2  InitialOutput=0
  "shifting, out" : Outport  Port=3  InitialOutput=0
  wires:
  gearbox speed estimator/1(Out1) -> MOTOR torque capability/1, downshift  command/3(engine speed), upshift  command/3(engine speed)
  gb_spd_in_r/1 -> gearbox speed estimator/1(gb_spd_in_r if no gear change)
  current gear number/1 -> Saturation1/1
  Saturation/1 -> Fcn/1
  prev. Pout/Pin/1 -> Saturation/1
  gb_trq_out_r/1 -> ~gb_trq_in_r/1
  upshift  command/1(command) -> delta gear number/1, delta gear number/2
  gear ratio/1 -> prev gear ratio/1
  Rate Limiter/1 -> gear ratio/1
  gb_spd_out_r/1 -> gb_spd_in_r/1
  downshift  command/1(command) -> Gain1/1
  Gain1/1 -> Product3/2
  Product3/1 -> delta gear number/3
  allow downshift?/1(allow shift) -> Product3/1
  prev gear ratio/1 -> Fcn1/1, gb_spd_in_r/2
  delta gear number/1 -> current gear number/2
  Fcn1/1 -> ~gb_trq_in_r/3
  MOTOR torque capability/1 -> Product2/2
  Product2/1 -> load=T/ (maxT at spd)/1
  ~gb_trq_in_r/1 -> Product2/1
  Fcn/1 -> ~gb_trq_in_r/2
  load=T/ (maxT at spd)/1 -> Switch/3
  tires are at traction limit/1 -> Switch/2
  Constant/1 -> Switch/1
  Switch/1 -> upshift  command/2(engine load), downshift  command/2(engine load)
  Saturation1/1 -> prev gear number/1, gear ratio1/1, shifting1/1(gear number), Rate Limiter/1, [def_gear_num]
  prev gear number/1 -> allow downshift?/1(prev gearnum), upshift  command/1(prev gear number), downshift  command/1(prev gear number), current gear number/1
  shifting1/1(out_1) -> [def_shifting]
  gear ratio1/1 -> [def_gear_ratio]
  Constant14/1 -> Switch3/2
  [def_gear_num] -> Switch3/3
  Constant15/1 -> Switch4/2
  [spd_dep_muxed] -> Switch4/1
  Mux/1 -> Switch4/3
  [def_gear_ratio] -> Mux/1
  [def_shifting] -> Mux/2
  Switch4/1 -> Demux/1
  [spd_dep_gear_num] -> Switch3/1
  [v_req_limited] -> Speed Dependent Shifting/1
  Speed Dependent Shifting/1 -> [spd_dep_muxed]
  Speed Dependent Shifting/2 -> [spd_dep_gear_num]
  Demux/1 -> "gear ratio, out"/1
  Demux/2 -> "shifting, out"/1
  Switch3/1 -> "gear number, out"/1

== system lib_controls/<vc> fuel cell/key_on ==
  Clock : Clock
  Fcn1 : Fcn  Expr=rem(u[1],period)
  Look-Up Table : Lookup  InputValues=t  Table=y  SaturateOnIntegerOverflow=on
  out_1 : Outport  InitialOutput=0
  wires:
  Look-Up Table/1 -> out_1/1
  Clock/1 -> Fcn1/1
  Fcn1/1 -> Look-Up Table/1

== system lib_controls/<vc> fuel cell/motor controller logic ==
  bus voltage : Inport
  req'd input power (W) : Inport  Port=2
  req'd output spd (rad/s) : Inport  Port=3
  shifting : Inport  Port=4
  Abs : Abs  SaturateOnIntegerOverflow=on
  Abs1 : Abs  SaturateOnIntegerOverflow=on
  Block NOTES : Subsystem
      mask Display: disp('Block\nNOTES')
  Constant : Constant  Value=mc_max_crrnt
  Constant1 : Constant  Value=0.001
  Constant2 : Constant  Value=0
  Logical Operator1 : Logic  Operator=NOT  Inputs=1
  Memory : Memory  X0=ess_module_num*mean(ess_voc(1,:))
  MinMax : MinMax  Inputs=2  SaturateOnIntegerOverflow=on  InputSameDT=on
  Product1 : Product  SaturateOnIntegerOverflow=on  RndMeth=Zero  InputSameDT=on  OutDataTypeStr=Inherit: Same as first input
  Relational Operator : RelationalOperator  Operator=<=  InputSameDT=on
  Relational Operator2 : RelationalOperator  Operator===  InputSameDT=on
  Sign : Subsystem
      mask Type: Sign
      mask Description: y = sign(x)
      mask Help: Sign Function:\n\t\t\ty = 1 if x > 0\n\t\t\ty = 0 if x = 0\n\t\t\ty = -1 if x < 0
      mask Display: plot(-50,-50,50,50,[-50,50],[0,0],[0,0],[-50,50],[-40,0],[-30,-30],[0,40],[30,30])
  Switch : Switch  Threshold=eps  SaturateOnIntegerOverflow=on  InputSameDT=on
  current-limited power : Product  SaturateOnIntegerOverflow=on  RndMeth=Zero  InputSameDT=on  OutDataTypeStr=Inherit: Same as first input
  true if motor should be shut down : Logic  Operator=OR
  req'd input power (W)1 : Outport  InitialOutput=0
  tag scope: mc_crrnt_limited=global
  wires:
  Abs1/1 -> Relational Operator/1
  true if motor should be shut down/1 -> Logical Operator1/1
  shifting/1 -> true if motor should be shut down/2
  Logical Operator1/1 -> Switch/2
  Constant/1 -> Product1/2
  Abs/1 -> MinMax/2
  Sign/1(out_1) -> current-limited power/2
  Constant2/1 -> Switch/3
  Switch/1 -> req'd input power (W)1/1
  current-limited power/1 -> Switch/1
  Product1/1 -> Relational Operator2/1, MinMax/1
  MinMax/1 -> current-limited power/1, Relational Operator2/2
  Relational Operator2/1 -> [mc_crrnt_limited]
  Relational Operator/1 -> true if motor should be shut down/1
  Constant1/1 -> Relational Operator/2
  req'd output spd (rad/s)/1 -> Abs1/1
  bus voltage/1 -> Memory/1
  Memory/1 -> Product1/1
  req'd input power (W)/1 -> Abs/1, Sign/1(in_1)

== system lib_controls/<vc> fuel cell/series 'clutch' control ==
  engine on : Inport
  Block NOTES : Subsystem
      mask Display: disp('Block\nNOTES')
  Clock : Clock
  Constant6 : Constant
  Constant7 : Constant  Value=3
  Memory1 : Memory  X0=cyc_mph(1,2)>0
  Memory2 : Memory  X0=-1
  Sum : Sum  Inputs=+-  SaturateOnIntegerOverflow=on  InputSameDT=on  OutDataTypeStr=Inherit: Same as first input
  Switch : Switch  Threshold=eps  SaturateOnIntegerOverflow=on  InputSameDT=on
  Switch1 : Switch  Threshold=0.5  SaturateOnIntegerOverflow=on  InputSameDT=on
  Transport Delay : TransportDelay  DelayTime=0.5
  clutch slipping1 : Logic
  clutch slipping2 : Logic
  clutch state : Outport
  wires:
  engine on/1 -> clutch slipping2/1, Transport Delay/1, Memory1/1, clutch slipping1/1
  Sum/1 -> Switch1/2
  Memory2/1 -> Sum/2
  Clock/1 -> Memory2/1, Sum/1
  clutch slipping2/1 -> Switch1/3
  Transport Delay/1 -> clutch slipping2/2
  clutch slipping1/1 -> Switch1/1
  Constant6/1 -> Switch/3
  Switch/1 -> clutch state/1
  Switch1/1 -> Switch/2
  Constant7/1 -> Switch/1
  Memory1/1 -> clutch slipping1/2

== system lib_controls/<vc> insight/config traction control ==
  time-average vehicle speed  req'd (m/s) : Inport
  vehicle speed at beginning of time  step (m/s) : Inport  Port=2
  total tractive force req'd (N) : Inport  Port=3
  traction control 2 axle : lib_controls/SubSystem/traction control 2 axle
      settings: RTWFcnNameOpts=Auto  RTWFileNameOpts=Auto
  req'd force (N) : Outport
  req'd speed (m/s) : Outport  Port=2
  weight on front axle (N) : Outport  Port=3
  weight on rear axle (N) : Outport  Port=4
  front/total  traction ratio : Outport  Port=5
  wires:
  time-average vehicle speed  req'd (m/s)/1 -> traction control 2 axle/1
  vehicle speed at beginning of time  step (m/s)/1 -> traction control 2 axle/2
  total tractive force req'd (N)/1 -> traction control 2 axle/3
  traction control 2 axle/1 -> req'd force (N)/1
  traction control 2 axle/2 -> req'd speed (m/s)/1
  traction control 2 axle/3 -> weight on front axle (N)/1
  traction control 2 axle/4 -> weight on rear axle (N)/1
  traction control 2 axle/5 -> front/total  traction ratio/1
